simulink model "krets4"  (R2017a)
settings: Solver=VariableStepAuto  StartTime=0.0  StopTime=0.0001  RelTol=1e-3
libraries: fl_lib x10, nesl_utility x6
settings Model: Creator=Caroline Skoglund  LastModifiedBy=Frans

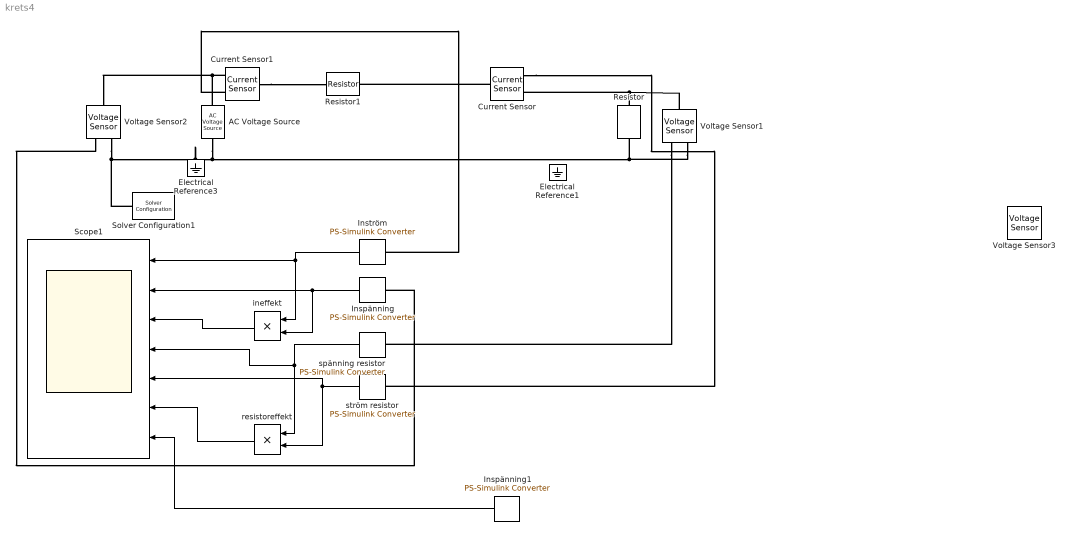
== system krets4 ==
  AC Voltage Source : fl_lib/Electrical/Electrical Sources/AC Voltage Source  amp=25 V  shift=0 deg  frequency=200 kHz  omega=0 rad/s
  Current Sensor : fl_lib/Electrical/Electrical Sensors/Current Sensor
  Current Sensor1 : fl_lib/Electrical/Electrical Sensors/Current Sensor
  Electrical Reference1 : fl_lib/Electrical/Electrical Elements/Electrical Reference
  Electrical Reference3 : fl_lib/Electrical/Electrical Elements/Electrical Reference
  Inspänning : nesl_utility/PS-Simulink Converter  PhysicalDomain=network_engine_domain  SubClassName=ps_output  LeftPortType=input  RightPortType=output  PseudoPeriodic=off  Frequencies=[]  Unit=1  AffineConversion=off
  Inspänning1 : nesl_utility/PS-Simulink Converter  PhysicalDomain=network_engine_domain  SubClassName=ps_output  LeftPortType=input  RightPortType=output  PseudoPeriodic=off  Frequencies=[]  Unit=1  AffineConversion=off
  Inström : nesl_utility/PS-Simulink Converter  PhysicalDomain=network_engine_domain  SubClassName=ps_output  LeftPortType=input  RightPortType=output  PseudoPeriodic=off  Frequencies=[]  Unit=1  AffineConversion=off
  Resistor : fl_lib/Electrical/Electrical Elements/Resistor  R=1.6570 Ohm  i_specify=off  i_priority=None  i=0 A  i_nominal_specify=off  i_nominal_unit=A  i_nominal_value=1  v_specify=off  v_priority=None  v=0 V  v_nominal_specify=off  v_nominal_unit=V  v_nominal_value=1
  Resistor1 : fl_lib/Electrical/Electrical Elements/Resistor  R=0.0775 Ohm  i_specify=off  i_priority=None  i=0 A  i_nominal_specify=off  i_nominal_unit=A  i_nominal_value=1  v_specify=off  v_priority=None  v=0 V  v_nominal_specify=off  v_nominal_unit=V  v_nominal_value=1
  Scope1 : Scope  NumInputPorts=7
  Solver Configuration1 : nesl_utility/Solver Configuration  PhysicalDomain=network_engine_domain  SubClassName=solver  LeftPortType=input  RightPortType=generic  Accelerate=off  Tones=[]  Harmonics=[]  SimulateNoise=off  Profile=off  UseLocalSampling=off  EnableSwitchedLinearOptims=on  FrequencyDomain=off  UseCCode=off  RelTol=0.001  AbsTol=1e-06  MinStep=1e-09  ToWorkspace=off  RevertToSquareIcSolve=off  NumHomotopyIterations=100  PhasorMode=off  PhasorModeNumHarmonics=1  OverrideAbsTol=off  DoDC=off  ResidualTolerance=1e-09  UseLocalSolver=off  LocalSolverChoice=NE_BACKWARD_EULER_ADVANCER  LocalSolverSampleTime=0.001  DoFixedCost=off  MaxNonlinIter=3  MaxModeIter=2  LinearAlgebra=Sparse  DelaysMemoryBudget=1024  AutomaticFiltering=on  FilteringTimeConstant=0.001
  Voltage Sensor1 : fl_lib/Electrical/Electrical Sensors/Voltage Sensor
  Voltage Sensor2 : fl_lib/Electrical/Electrical Sensors/Voltage Sensor
  Voltage Sensor3 : fl_lib/Electrical/Electrical Sensors/Voltage Sensor
  ineffekt : Product
  resistoreffekt : Product
  spänning resistor : nesl_utility/PS-Simulink Converter  PhysicalDomain=network_engine_domain  SubClassName=ps_output  LeftPortType=input  RightPortType=output  PseudoPeriodic=off  Frequencies=[]  Unit=1  AffineConversion=off
  ström resistor : nesl_utility/PS-Simulink Converter  PhysicalDomain=network_engine_domain  SubClassName=ps_output  LeftPortType=input  RightPortType=output  PseudoPeriodic=off  Frequencies=[]  Unit=1  AffineConversion=off
  wires:
  spänning resistor/1 -> resistoreffekt/1, Scope1/4
  ström resistor/1 -> resistoreffekt/2, Scope1/5
  resistoreffekt/1 -> Scope1/6
  Inspänning/1 -> ineffekt/2, Scope1/2
  Inström/1 -> ineffekt/1, Scope1/1
  ineffekt/1 -> Scope1/3
  Inspänning1/1 -> Scope1/7
  connections:
  Solver Configuration1/RConn1 -- Voltage Sensor2/RConn2 -- Electrical Reference3/LConn1 -- Voltage Sensor1/RConn2 -- Resistor/RConn1 -- AC Voltage Source/RConn1
  Voltage Sensor1/RConn1 -- spänning resistor/LConn1
  Current Sensor/RConn1 -- ström resistor/LConn1
  Voltage Sensor2/RConn1 -- Inspänning/LConn1
  Resistor/LConn1 -- Voltage Sensor1/LConn1 -- Current Sensor/RConn2
  AC Voltage Source/LConn1 -- Voltage Sensor2/LConn1 -- Current Sensor1/RConn2
  Current Sensor1/RConn1 -- Inström/LConn1
  Current Sensor/LConn1 -- Resistor1/RConn1
  Current Sensor1/LConn1 -- Resistor1/LConn1
